simulink model "InductionCookerStateFlow_HarnessInductionCookerS6"  (R2023a)
settings: Solver=FixedStepDiscrete  StartTime=0.0  StopTime=2000  FixedStep=0.1  RelTol=1e-3  EnableMultiTasking=on
settings Model: Creator=antonio  LastModifiedBy=anton
settings SolverCC: AlgebraicLoopSolver=TrustRegion  AutoInsertRateTranBlk=on
settings DataIOCC: LimitDataPoints=on
settings OptimizationCC: LifeSpan=inf
settings DebuggingCC: UnconnectedInputMsg=warning  UnconnectedOutputMsg=warning  UnconnectedLineMsg=warning  AllowSymbolicDim=off  SFUnexpectedBacktrackingDiag=warning  SFNoUnconditionalDefaultTransitionDiag=warning  SFExecutionAtInitializationDiag=none  ArithmeticOperatorsInVariantConditions=warning
settings ModelReferenceCC: EnableRefExpFcnMdlSchedulingChecks=on
settings SFSimCC: SimUseLocalCustomCode=off  CustomCodeUndefinedFunction=UseInterfaceOnly
settings RTWCC: RTWUseLocalCustomCode=off  DLArmComputeVersion=19.05
settings CodeAppCC: StateflowObjectComments=on
settings GRTTargetCC: TargetLangStandard=C89/C90 (ANSI)
settings ConfigComp: CovEnable=on  RecordCoverage=on  CovMetricSettings=dw  CovSaveCumulativeToWorkspaceVar=on  CovSaveSingleToWorkspaceVar=on  CovModelRefEnable=on

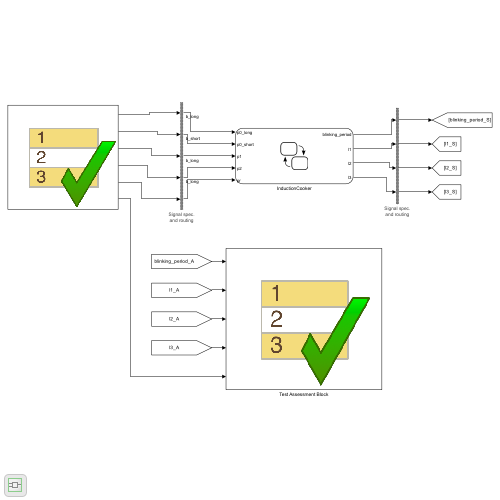
[thumbnail: Simulink's stored preview of the top-level diagram]
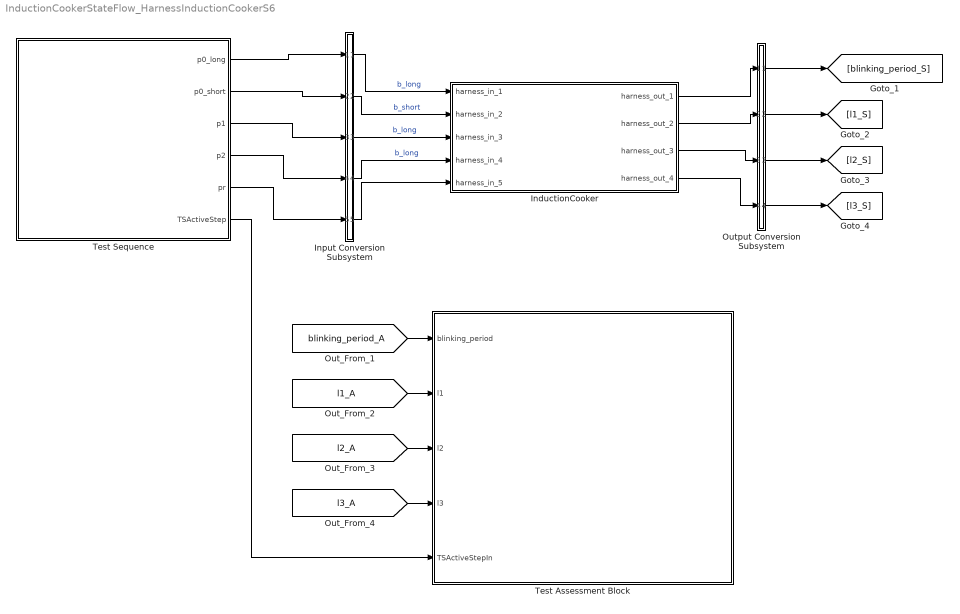
== system InductionCookerStateFlow_HarnessInductionCookerS6 ==
  InductionCooker : Subsystem  Tag=__SL_testing_harness_stub_
  Input Conversion Subsystem : Subsystem  Tag=__SLT_ICS__  Description=|
      | Signal spec.
      | and routing
      settings: AttributesFormatString=%<Description>
  Output Conversion Subsystem : Subsystem  Tag=__SLT_OCS__  Description=|
      | Signal spec.
      | and routing
      settings: AttributesFormatString=%<Description>
  Test Assessment Block : Test Sequence  Tag=__SLT_ASMT__  TreatAsAtomicUnit=on
  Test Sequence : Test Sequence  TreatAsAtomicUnit=on
  wires:
  [blinking_period_A] -> Test Assessment Block/1(blinking_period)
  [l1_A] -> Test Assessment Block/2(l1)
  [l2_A] -> Test Assessment Block/3(l2)
  [l3_A] -> Test Assessment Block/4(l3)
  Test Sequence/1(p0_long) -> Input Conversion Subsystem/1(Inport_1)
  Test Sequence/2(p0_short) -> Input Conversion Subsystem/2(Inport_2)
  Test Sequence/3(p1) -> Input Conversion Subsystem/3(Inport_3)
  Test Sequence/4(p2) -> Input Conversion Subsystem/4(Inport_4)
  Test Sequence/5(pr) -> Input Conversion Subsystem/5(Inport_5)
  Output Conversion Subsystem/1(Outport_1) -> [blinking_period_S]
  Output Conversion Subsystem/2(Outport_2) -> [l1_S]
  Output Conversion Subsystem/3(Outport_3) -> [l2_S]
  Output Conversion Subsystem/4(Outport_4) -> [l3_S]
  Test Sequence/6(TSActiveStep) -> Test Assessment Block/5(TSActiveStepIn)
  InductionCooker/1(harness_out_1) -> Output Conversion Subsystem/1(Inport_1)
  InductionCooker/2(harness_out_2) -> Output Conversion Subsystem/2(Inport_2)
  InductionCooker/3(harness_out_3) -> Output Conversion Subsystem/3(Inport_3)
  InductionCooker/4(harness_out_4) -> Output Conversion Subsystem/4(Inport_4)
  Input Conversion Subsystem/1(Outport_1) -> InductionCooker/1(harness_in_1)  "b_long"
  Input Conversion Subsystem/2(Outport_2) -> InductionCooker/2(harness_in_2)  "b_short"
  Input Conversion Subsystem/3(Outport_3) -> InductionCooker/3(harness_in_3)  "b_long"
  Input Conversion Subsystem/4(Outport_4) -> InductionCooker/4(harness_in_4)  "b_long"
  Input Conversion Subsystem/5(Outport_5) -> InductionCooker/5(harness_in_5)

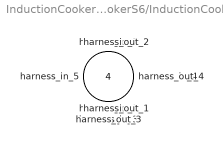
== system InductionCookerStateFlow_HarnessInductionCookerS6/InductionCooker ==
  harness_in_1 : Inport
  harness_in_2 : Inport  Port=2
  harness_in_3 : Inport  Port=3
  harness_in_4 : Inport  Port=4
  harness_in_5 : Inport  Port=5
  harness_out_1 : Outport
  harness_out_2 : Outport  Port=2
  harness_out_3 : Outport  Port=3
  harness_out_4 : Outport  Port=4

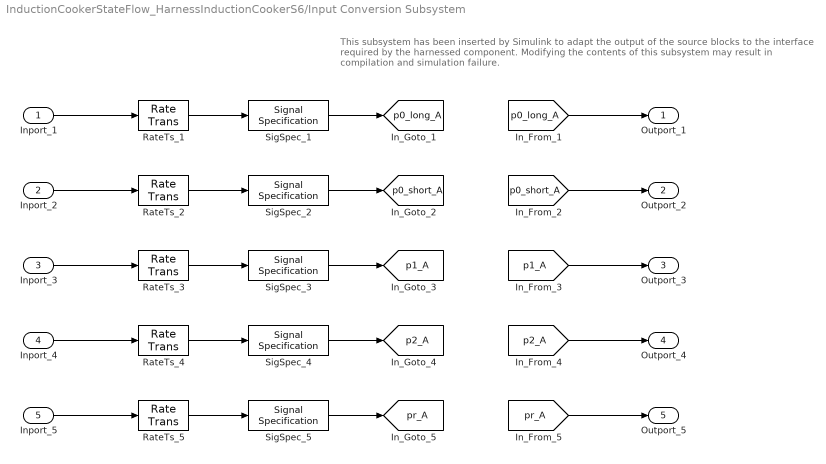
== system InductionCookerStateFlow_HarnessInductionCookerS6/Input Conversion Subsystem ==
  note: This subsystem has been inserted by Simulink to adapt the output of the source blocks to the interface required by the harnessed component.
      |  Modifying the contents of this subsystem may result in compilation and simulation failure.
  Inport_1 : Inport
  Inport_2 : Inport  Port=2
  Inport_3 : Inport  Port=3
  Inport_4 : Inport  Port=4
  Inport_5 : Inport  Port=5
  RateTs_{1..5} (5 alike) : RateTransition  OutPortSampleTime=0.1
  SigSpec_{1..5} (5 alike) : SignalSpecification  OutDataTypeStr=boolean  Dimensions=[1]  SampleTime=0.1
  Outport_1 : Outport
  Outport_2 : Outport  Port=2
  Outport_3 : Outport  Port=3
  Outport_4 : Outport  Port=4
  Outport_5 : Outport  Port=5
  tag scope: p0_long_A=global, p0_short_A=global, p1_A=global, p2_A=global, pr_A=global
  wires:
  [p0_long_A] -> Outport_1/1
  SigSpec_1/1 -> [p0_long_A]
  RateTs_1/1 -> SigSpec_1/1
  Inport_1/1 -> RateTs_1/1
  [p0_short_A] -> Outport_2/1
  SigSpec_2/1 -> [p0_short_A]
  RateTs_2/1 -> SigSpec_2/1
  Inport_2/1 -> RateTs_2/1
  [p1_A] -> Outport_3/1
  SigSpec_3/1 -> [p1_A]
  RateTs_3/1 -> SigSpec_3/1
  Inport_3/1 -> RateTs_3/1
  [p2_A] -> Outport_4/1
  SigSpec_4/1 -> [p2_A]
  RateTs_4/1 -> SigSpec_4/1
  Inport_4/1 -> RateTs_4/1
  [pr_A] -> Outport_5/1
  SigSpec_5/1 -> [pr_A]
  RateTs_5/1 -> SigSpec_5/1
  Inport_5/1 -> RateTs_5/1

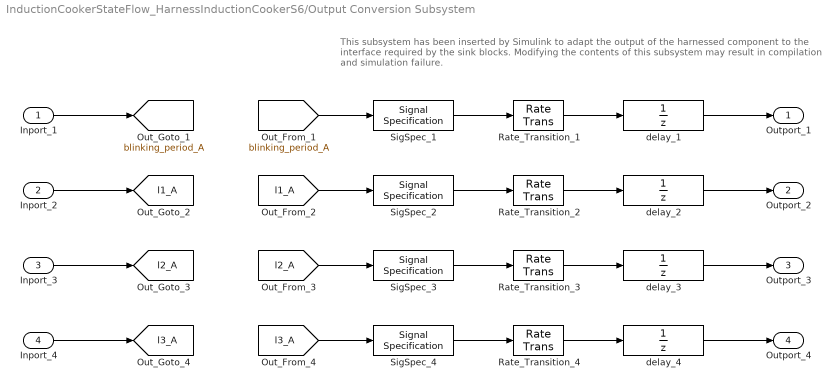
== system InductionCookerStateFlow_HarnessInductionCookerS6/Output Conversion Subsystem ==
  note: This subsystem has been inserted by Simulink to adapt the output of the harnessed component to the interface required by the sink blocks.
      |  Modifying the contents of this subsystem may result in compilation and simulation failure.
  Inport_1 : Inport
  Inport_2 : Inport  Port=2
  Inport_3 : Inport  Port=3
  Inport_4 : Inport  Port=4
  Rate_Transition_{1..4} (4 alike) : RateTransition  OutPortSampleTimeOpt=Inherit
  SigSpec_1 : SignalSpecification  OutDataTypeStr=uint32  Dimensions=[1]  SampleTime=0.1
  SigSpec_2 : SignalSpecification  OutDataTypeStr=boolean  Dimensions=[1]  SampleTime=0.1
  SigSpec_3 : SignalSpecification  OutDataTypeStr=boolean  Dimensions=[1]  SampleTime=0.1
  SigSpec_4 : SignalSpecification  OutDataTypeStr=boolean  Dimensions=[1]  SampleTime=0.1
  delay_{1..4} (4 alike) : UnitDelay  SampleTime=-1
  Outport_1 : Outport
  Outport_2 : Outport  Port=2
  Outport_3 : Outport  Port=3
  Outport_4 : Outport  Port=4
  tag scope: blinking_period_A=global, l1_A=global, l2_A=global, l3_A=global
  wires:
  Inport_1/1 -> [blinking_period_A]
  [blinking_period_A] -> SigSpec_1/1
  SigSpec_1/1 -> Rate_Transition_1/1
  Rate_Transition_1/1 -> delay_1/1
  delay_1/1 -> Outport_1/1
  Inport_2/1 -> [l1_A]
  [l1_A] -> SigSpec_2/1
  SigSpec_2/1 -> Rate_Transition_2/1
  Rate_Transition_2/1 -> delay_2/1
  delay_2/1 -> Outport_2/1
  Inport_3/1 -> [l2_A]
  [l2_A] -> SigSpec_3/1
  SigSpec_3/1 -> Rate_Transition_3/1
  Rate_Transition_3/1 -> delay_3/1
  delay_3/1 -> Outport_3/1
  Inport_4/1 -> [l3_A]
  [l3_A] -> SigSpec_4/1
  SigSpec_4/1 -> Rate_Transition_4/1
  Rate_Transition_4/1 -> delay_4/1
  delay_4/1 -> Outport_4/1

== stateflow chart InductionCookerStateFlow_HarnessInductionCookerS6/Test Assessment Block ==
  state Scenario_1
    state Run
      state VerifyInitS6
        verify(blinking_period == 0 & ~l1 & ~l2 & ~l3)
      state VerifyOnWithPotPresentS6
        verify(blinking_period == 0 & l1 & ~l2 & ~l3)
      state VerifyInactiveWithPotPresentS6
        verify(blinking_period == 0 & l1 & ~l2 & ~l3)
      state VerifyPowerIncreaseWithPotPresentS6
        verify(blinking_period == 0 & l1 & ~l2 & ~l3)
      state VerifyActive300WS6
        verify(blinking_period == 2000 & l1 & l2 & ~l3)
      state VerifyPowerIncreaseWithPotPresentAgainS6
        verify(blinking_period == 2000 & l1 & l2 & ~l3)
      state VerifyActive500WS6
        verify(blinking_period == 1000 & l1 & l2 & ~l3)
      state VerifyLongPressOffWithPotPresentS6
        verify(blinking_period == 0 & ~l1 & ~l2 & ~l3)
      state VerifyReleaseOffS6
        verify(blinking_period == 0 & ~l1 & ~l2 & ~l3)
      state step_1_2
      (default) -> (junction 795)
      Run -> (junction 795)
      (junction 795) -> (junction 796) [order 1] : [TSActiveStepIn == TSActiveStepEnumHInductionCooker.InitS6
          | ]
      (junction 796) -> VerifyInitS6 [order 1] : [~in(Scenario_1.Run.VerifyInitS6)]
      (junction 795) -> (junction 805) [order 2]
      (junction 796) -> (junction 799) [order 2]
      (junction 805) -> (junction 806) [order 1] : [TSActiveStepIn == TSActiveStepEnumHInductionCooker.OnWithPotPresentS6
          | ]
      (junction 806) -> VerifyOnWithPotPresentS6 [order 1] : [~in(Scenario_1.Run.VerifyOnWithPotPresentS6)]
      (junction 805) -> (junction 813) [order 2]
      (junction 806) -> (junction 809) [order 2]
      (junction 813) -> (junction 814) [order 1] : [TSActiveStepIn == TSActiveStepEnumHInductionCooker.InactiveWithPotPresentS6
          | ]
      (junction 814) -> VerifyInactiveWithPotPresentS6 [order 1] : [~in(Scenario_1.Run.VerifyInactiveWithPotPresentS6)]
      (junction 813) -> (junction 821) [order 2]
      (junction 814) -> (junction 817) [order 2]
      (junction 821) -> (junction 822) [order 1] : [TSActiveStepIn == TSActiveStepEnumHInductionCooker.PowerIncreaseWithPotPresentS6
          | ]
      (junction 822) -> VerifyPowerIncreaseWithPotPresentS6 [order 1] : [~in(Scenario_1.Run.VerifyPowerIncreaseWithPotPresentS6)]
      (junction 821) -> (junction 837) [order 2]
      (junction 822) -> (junction 825) [order 2]
      (junction 837) -> (junction 838) [order 1] : [TSActiveStepIn == TSActiveStepEnumHInductionCooker.Active300WS6
          | ]
      (junction 838) -> VerifyActive300WS6 [order 1] : [~in(Scenario_1.Run.VerifyActive300WS6)]
      (junction 837) -> (junction 873) [order 2]
      (junction 838) -> (junction 841) [order 2]
      (junction 873) -> (junction 874) [order 1] : [TSActiveStepIn == TSActiveStepEnumHInductionCooker.PowerIncreaseWithPotPresentAgainS6
          | ]
      (junction 874) -> VerifyPowerIncreaseWithPotPresentAgainS6 [order 1] : [~in(Scenario_1.Run.VerifyPowerIncreaseWithPotPresentAgainS6)]
      (junction 882) -> (junction 845) [order 2]
      (junction 874) -> (junction 877) [order 2]
      (junction 882) -> (junction 883) [order 1] : [TSActiveStepIn == TSActiveStepEnumHInductionCooker.Active500WS6
          | ]
      (junction 883) -> VerifyActive500WS6 [order 1] : [~in(Scenario_1.Run.VerifyActive500WS6)]
      (junction 845) -> (junction 846) [order 1] : [TSActiveStepIn == TSActiveStepEnumHInductionCooker.LongPressOffWithPotPresentS6
          | ]
      (junction 846) -> VerifyLongPressOffWithPotPresentS6 [order 1] : [~in(Scenario_1.Run.VerifyLongPressOffWithPotPresentS6)]
      (junction 845) -> (junction 853) [order 2]
      (junction 846) -> (junction 849) [order 2]
      (junction 853) -> (junction 854) [order 1] : [TSActiveStepIn == TSActiveStepEnumHInductionCooker.ReleaseOffS6
          | ]
      (junction 854) -> VerifyReleaseOffS6 [order 1] : [~in(Scenario_1.Run.VerifyReleaseOffS6)]
      (junction 853) -> (junction 861) [order 2]
      (junction 854) -> (junction 857) [order 2]
      (junction 861) -> (junction 862)
      (junction 862) -> step_1_2 [order 1] : [~in(Scenario_1.Run.step_1_2)]
      (junction 862) -> (junction 865) [order 2]
      (junction 883) -> (junction 886) [order 2]
      (junction 873) -> (junction 882) [order 2]
    (default) -> Run
  (default) -> Scenario_1 : {assert(Active_Scenario_Index == 1,'The value of Scenario Parameter ''Active_Scenario_Index'' is not valid. Use the index of the scenario to specify it.')}
  data: blinking_period input uint32 size=[1]; l1 input boolean size=[1]; l2 input boolean size=[1]; l3 input boolean size=[1]; TSActiveStepIn input; Active_Scenario_Index parameter =1

== stateflow chart InductionCookerStateFlow_HarnessInductionCookerS6/Test Sequence ==
  settings: updateMethod=DISCRETE  sampleTime=0.1
  state Scenario_1
    state InitS6
      p0_long = true;
      p0_short = true;
      p1 = true;
      p2 = true;
      pr = false;
      settings: description=|
          | Condizione in cui tutti i pulsanti sono rilasciati e
          | la pentola è presente sul dispositivo.
    state OnWithPotPresentS6
      p0_long = true;
      p0_short = false;
      p1 = true;
      p2 = true;
      pr = false;
      settings: description=|
          | Condizione in cui il pulsante per l'accensione è
          | premuto, mentre tutti gli altri pulsanti sono
          | rilasciati e la pentola è presente sul dispositivo.
    state InactiveWithPotPresentS6
      p0_long = true;
      p0_short = true;
      p1 = true;
      p2 = true;
      pr = false;
      settings: description=|
          | Condizione in cui tutti i pulsanti sono rilasciati e la
          | pentola è presente sul dispositivo.
    state PowerIncreaseWithPotPresentS6
      p0_long = true;
      p0_short = true;
      p1 = false;
      p2 = true;
      pr =  false;
      settings: description=|
          | Condizione in cui il pulsante per l'aumento della
          | potenza è premuto per almeno 1 secondo, mentre
          | tutti gli altri pulsanti sono rilasciati e la pentola è
          | presente sul dispositivo.
    state Waiting300WS6
      p0_long = true;
      p0_short = true;
      p1 = true;
      p2 = true;
      pr =  false;
      settings: description=|
          | Condizione in cui tutti i pulsanti sono rilasciati
          | e la pentola è presente sul dispositivo.
          | Si attende che passino i 5 secondi per
          | l'effettivo cambio della potenza.
    state Active300WS6
      p0_long = true;
      p0_short = true;
      p1 = true;
      p2 = true;
      pr =  false;
      settings: description=|
          | Condizione in cui tutti i pulsanti sono rilasciati, la
          | pentola è presente sul dispositivo e quest'ultimo sta
          | erogando la potenza desiderata.
    state PowerIncreaseWithPotPresentAgainS6
      p0_long = true;
      p0_short = true;
      p1 = false;
      p2 = true;
      pr =  false;
      settings: description=|
          | Condizione in cui il pulsante per l'aumento della
          | potenza è premuto per almeno 1 secondo, mentre
          | tutti gli altri pulsanti sono rilasciati e la pentola è
          | presente sul dispositivo.
    state Waiting500WS6
      p0_long = true;
      p0_short = true;
      p1 = true;
      p2 = true;
      pr =  false;
      settings: description=|
          | Condizione in cui tutti i pulsanti sono rilasciati
          | e la pentola è presente sul dispositivo.
          | Si attende che passino i 5 secondi per
          | l'effettivo cambio della potenza.
    state Active500WS6
      p0_long = true;
      p0_short = true;
      p1 = true;
      p2 = true;
      pr =  false;
      settings: description=|
          | Condizione in cui si sta erogando la potenza
          | selezionata.
    state LongPressOffWithPotPresentS6
      p0_long = false;
      p0_short = true;
      p1 = true;
      p2 = true;
      pr =  false;
      settings: description=|
          | Condizione in cui il pulsante per lo spegnimento
          | è premuto per almeno 1 secondo, mentre tutti gli
          | altri pulsanti sono rilasciati e la pentola è presente
          | sul dispositivo.
    state ReleaseOffS6
      p0_long = true;
      p0_short = true;
      p1 = true;
      p2 = true;
      pr =  false;
      settings: description=|
          | Ritorno alla condizione iniziale rilasciando il
          | pulsante di spegnimento.
    (default) -> InitS6
    InitS6 -> OnWithPotPresentS6 : [
        | true
        | ]
    OnWithPotPresentS6 -> InactiveWithPotPresentS6 : [
        | true
        | ]
    InactiveWithPotPresentS6 -> PowerIncreaseWithPotPresentS6 : [
        | true
        | ]
    PowerIncreaseWithPotPresentS6 -> Waiting300WS6 : [
        | true
        | ]
    Waiting300WS6 -> Active300WS6 : [
        | after(5, sec)
        | ]
    Active300WS6 -> PowerIncreaseWithPotPresentAgainS6 : [
        | true
        | ]
    PowerIncreaseWithPotPresentAgainS6 -> Waiting500WS6 : [
        | true
        | ]
    Waiting500WS6 -> Active500WS6 : [
        | after(5, sec)
        | ]
    Active500WS6 -> LongPressOffWithPotPresentS6 : [
        | after(8, sec)
        | ]
    LongPressOffWithPotPresentS6 -> ReleaseOffS6 : [
        | true
        | ]
  (default) -> Scenario_1 : {assert(Active_Scenario_Index == 1,'The value of Scenario Parameter ''Active_Scenario_Index'' is not valid. Use the index of the scenario to specify it.')}
  data: p0_long output boolean size=[1]; p0_short output boolean size=[1]; p1 output boolean size=[1]; p2 output boolean size=[1]; pr output boolean size=[1]; TSActiveStep output Enum: TSActiveStepEnumHInductionCooker; Active_Scenario_Index parameter =1
